simulink model "ejemplo_arduino2"  (R2014b)
settings: Solver=ode3  StartTime=0.0  StopTime=inf  FixedStep=0.001  RelTol=1e-3
libraries: simulink x48, simulink_extras x36, dspswit3 x16, LibrarySimulinkSAS x2, vrlib x2, sldrtlib x1
(part 2 of 2)

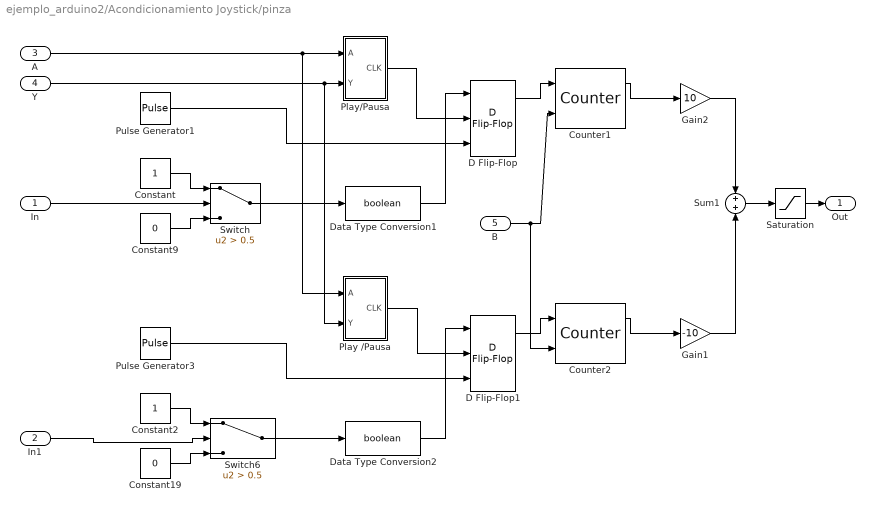
== system ejemplo_arduino2/Acondicionamiento Joystick/pinza ==
  In : Inport
  In1 : Inport  Port=2
  A : Inport  Port=3
  Y : Inport  Port=4
  B : Inport  Port=5
  Constant : Constant
  Constant19 : Constant  Value=0
  Constant2 : Constant
  Constant9 : Constant  Value=0
  Counter1 : dspswit3/Counter  Direction=Up  CountEvent=Rising edge  CounterSize=User defined  MaxCount=255  InitialCount=0  Output=Count and Hit  HitValue=32  ResetInput=on  SamplesPerFrame=1  Ts=1  CntDtype=double  HitDtype=Logical
  Counter2 : dspswit3/Counter  Direction=Up  CountEvent=Rising edge  CounterSize=User defined  MaxCount=255  InitialCount=0  Output=Count and Hit  HitValue=32  ResetInput=on  SamplesPerFrame=1  Ts=1  CntDtype=double  HitDtype=Logical
  D Flip-Flop : simulink_extras/Flip Flops/D Flip-Flop
  D Flip-Flop1 : simulink_extras/Flip Flops/D Flip-Flop
  Data Type Conversion1 : DataTypeConversion  OutDataTypeStr=boolean
  Data Type Conversion2 : DataTypeConversion  OutDataTypeStr=boolean
  Gain1 : Gain  Gain=-10
  Gain2 : Gain  Gain=10
  Play /Pausa : Subsystem
  Play/Pausa : Subsystem
  Pulse Generator1 : DiscretePulseGenerator  PulseType=Time based  Period=0.1  PulseWidth=50
  Pulse Generator3 : DiscretePulseGenerator  PulseType=Time based  Period=0.1  PulseWidth=50
  Saturation : Saturate  UpperLimit=200  LowerLimit=0
  Sum1 : Sum  Inputs=+|+
  Switch : Switch  Criteria=u2 > Threshold  Threshold=0.5  OutDataTypeStr=single  InputSameDT=on
  Switch6 : Switch  Criteria=u2 > Threshold  Threshold=0.5  OutDataTypeStr=single  InputSameDT=on
  Out : Outport
  wires:
  Counter1/1 -> Gain2/1
  Constant/1 -> Switch/1
  Constant9/1 -> Switch/3
  Constant2/1 -> Switch6/1
  Counter2/1 -> Gain1/1
  Gain1/1 -> Sum1/2
  D Flip-Flop1/1 -> Counter2/1
  Switch6/1 -> Data Type Conversion2/1
  Data Type Conversion2/1 -> D Flip-Flop1/1
  Pulse Generator3/1 -> D Flip-Flop1/3
  Constant19/1 -> Switch6/3
  In/1 -> Switch/2
  Saturation/1 -> Out/1
  Pulse Generator1/1 -> D Flip-Flop/3
  Sum1/1 -> Saturation/1
  Gain2/1 -> Sum1/1
  D Flip-Flop/1 -> Counter1/1
  Data Type Conversion1/1 -> D Flip-Flop/1
  Switch/1 -> Data Type Conversion1/1
  In1/1 -> Switch6/2
  Play/Pausa/1(CLK) -> D Flip-Flop/2
  Play /Pausa/1(CLK) -> D Flip-Flop1/2
  A/1 -> Play /Pausa/1(A), Play/Pausa/1(A)
  Y/1 -> Play /Pausa/2(Y), Play/Pausa/2(Y)
  B/1 -> Counter1/2, Counter2/2

== system ejemplo_arduino2/Acondicionamiento Joystick/Horizontal/Play //Pausa ==
  A : Inport
  Y : Inport  Port=2
  Constant1 : Constant  Value=0
  Detect Rise Positive : simulink/Logic and Bit Operations/Detect Rise Positive  vinit=0  InputProcessing=Inherited  OutDataTypeStr=boolean
  Detect Rise Positive1 : simulink/Logic and Bit Operations/Detect Rise Positive  vinit=0  InputProcessing=Inherited  OutDataTypeStr=boolean
  Pulse Generator : DiscretePulseGenerator  PulseType=Time based  Period=0.05  PulseWidth=50
  S-R Flip-Flop : simulink_extras/Flip Flops/S-R Flip-Flop  initial_condition=0
  Switch1 : Switch  Criteria=u2 > Threshold  Threshold=0.5  OutDataTypeStr=single  InputSameDT=on
  CLK : Outport
  wires:
  Pulse Generator/1 -> Switch1/1
  S-R Flip-Flop/1 -> Switch1/2
  Switch1/1 -> CLK/1
  Constant1/1 -> Switch1/3
  Detect Rise Positive1/1 -> S-R Flip-Flop/2
  A/1 -> Detect Rise Positive/1
  Detect Rise Positive/1 -> S-R Flip-Flop/1
  Y/1 -> Detect Rise Positive1/1

== system ejemplo_arduino2/Acondicionamiento Joystick/Horizontal/Play//Pausa ==
  A : Inport
  Y : Inport  Port=2
  Constant1 : Constant  Value=0
  Detect Rise Positive : simulink/Logic and Bit Operations/Detect Rise Positive  vinit=0  InputProcessing=Inherited  OutDataTypeStr=boolean
  Detect Rise Positive1 : simulink/Logic and Bit Operations/Detect Rise Positive  vinit=0  InputProcessing=Inherited  OutDataTypeStr=boolean
  Pulse Generator : DiscretePulseGenerator  PulseType=Time based  Period=0.05  PulseWidth=50
  S-R Flip-Flop : simulink_extras/Flip Flops/S-R Flip-Flop  initial_condition=0
  Switch1 : Switch  Criteria=u2 > Threshold  Threshold=0.5  OutDataTypeStr=single  InputSameDT=on
  CLK : Outport
  wires:
  Pulse Generator/1 -> Switch1/1
  S-R Flip-Flop/1 -> Switch1/2
  Switch1/1 -> CLK/1
  Constant1/1 -> Switch1/3
  Detect Rise Positive1/1 -> S-R Flip-Flop/2
  A/1 -> Detect Rise Positive/1
  Detect Rise Positive/1 -> S-R Flip-Flop/1
  Y/1 -> Detect Rise Positive1/1

== system ejemplo_arduino2/Acondicionamiento Joystick/Vertical/Play //Pausa ==
  A : Inport
  Y : Inport  Port=2
  Constant1 : Constant  Value=0
  Detect Rise Positive : simulink/Logic and Bit Operations/Detect Rise Positive  vinit=0  InputProcessing=Inherited  OutDataTypeStr=boolean
  Detect Rise Positive1 : simulink/Logic and Bit Operations/Detect Rise Positive  vinit=0  InputProcessing=Inherited  OutDataTypeStr=boolean
  Pulse Generator : DiscretePulseGenerator  PulseType=Time based  Period=0.1  PulseWidth=50
  S-R Flip-Flop : simulink_extras/Flip Flops/S-R Flip-Flop  initial_condition=0
  Switch1 : Switch  Criteria=u2 > Threshold  Threshold=0.5  OutDataTypeStr=single  InputSameDT=on
  CLK : Outport
  wires:
  Pulse Generator/1 -> Switch1/1
  S-R Flip-Flop/1 -> Switch1/2
  Switch1/1 -> CLK/1
  Constant1/1 -> Switch1/3
  Detect Rise Positive1/1 -> S-R Flip-Flop/2
  A/1 -> Detect Rise Positive/1
  Detect Rise Positive/1 -> S-R Flip-Flop/1
  Y/1 -> Detect Rise Positive1/1

== system ejemplo_arduino2/Acondicionamiento Joystick/Vertical/Play//Pausa ==
  A : Inport
  Y : Inport  Port=2
  Constant1 : Constant  Value=0
  Detect Rise Positive : simulink/Logic and Bit Operations/Detect Rise Positive  vinit=0  InputProcessing=Inherited  OutDataTypeStr=boolean
  Detect Rise Positive1 : simulink/Logic and Bit Operations/Detect Rise Positive  vinit=0  InputProcessing=Inherited  OutDataTypeStr=boolean
  Pulse Generator : DiscretePulseGenerator  PulseType=Time based  Period=0.1  PulseWidth=50
  S-R Flip-Flop : simulink_extras/Flip Flops/S-R Flip-Flop  initial_condition=0
  Switch1 : Switch  Criteria=u2 > Threshold  Threshold=0.5  OutDataTypeStr=single  InputSameDT=on
  CLK : Outport
  wires:
  Pulse Generator/1 -> Switch1/1
  S-R Flip-Flop/1 -> Switch1/2
  Switch1/1 -> CLK/1
  Constant1/1 -> Switch1/3
  Detect Rise Positive1/1 -> S-R Flip-Flop/2
  A/1 -> Detect Rise Positive/1
  Detect Rise Positive/1 -> S-R Flip-Flop/1
  Y/1 -> Detect Rise Positive1/1

== system ejemplo_arduino2/Acondicionamiento Joystick/mov 1/Play //Pausa ==
  A : Inport
  Y : Inport  Port=2
  Constant1 : Constant  Value=0
  Detect Rise Positive : simulink/Logic and Bit Operations/Detect Rise Positive  vinit=0  InputProcessing=Inherited  OutDataTypeStr=boolean
  Detect Rise Positive1 : simulink/Logic and Bit Operations/Detect Rise Positive  vinit=0  InputProcessing=Inherited  OutDataTypeStr=boolean
  Pulse Generator : DiscretePulseGenerator  PulseType=Time based  Period=0.1  PulseWidth=50
  S-R Flip-Flop : simulink_extras/Flip Flops/S-R Flip-Flop  initial_condition=0
  Switch1 : Switch  Criteria=u2 > Threshold  Threshold=0.5  OutDataTypeStr=single  InputSameDT=on
  CLK : Outport
  wires:
  Pulse Generator/1 -> Switch1/1
  S-R Flip-Flop/1 -> Switch1/2
  Switch1/1 -> CLK/1
  Constant1/1 -> Switch1/3
  Detect Rise Positive1/1 -> S-R Flip-Flop/2
  A/1 -> Detect Rise Positive/1
  Detect Rise Positive/1 -> S-R Flip-Flop/1
  Y/1 -> Detect Rise Positive1/1

== system ejemplo_arduino2/Acondicionamiento Joystick/mov 1/Play//Pausa ==
  A : Inport
  Y : Inport  Port=2
  Constant1 : Constant  Value=0
  Detect Rise Positive : simulink/Logic and Bit Operations/Detect Rise Positive  vinit=0  InputProcessing=Inherited  OutDataTypeStr=boolean
  Detect Rise Positive1 : simulink/Logic and Bit Operations/Detect Rise Positive  vinit=0  InputProcessing=Inherited  OutDataTypeStr=boolean
  Pulse Generator : DiscretePulseGenerator  PulseType=Time based  Period=0.1  PulseWidth=50
  S-R Flip-Flop : simulink_extras/Flip Flops/S-R Flip-Flop  initial_condition=0
  Switch1 : Switch  Criteria=u2 > Threshold  Threshold=0.5  OutDataTypeStr=single  InputSameDT=on
  CLK : Outport
  wires:
  Pulse Generator/1 -> Switch1/1
  S-R Flip-Flop/1 -> Switch1/2
  Switch1/1 -> CLK/1
  Constant1/1 -> Switch1/3
  Detect Rise Positive1/1 -> S-R Flip-Flop/2
  A/1 -> Detect Rise Positive/1
  Detect Rise Positive/1 -> S-R Flip-Flop/1
  Y/1 -> Detect Rise Positive1/1

== system ejemplo_arduino2/Acondicionamiento Joystick/mov 2/Play //Pausa ==
  A : Inport
  Y : Inport  Port=2
  Constant1 : Constant  Value=0
  Detect Rise Positive : simulink/Logic and Bit Operations/Detect Rise Positive  vinit=0  InputProcessing=Inherited  OutDataTypeStr=boolean
  Detect Rise Positive1 : simulink/Logic and Bit Operations/Detect Rise Positive  vinit=0  InputProcessing=Inherited  OutDataTypeStr=boolean
  Pulse Generator : DiscretePulseGenerator  PulseType=Time based  Period=0.1  PulseWidth=50
  S-R Flip-Flop : simulink_extras/Flip Flops/S-R Flip-Flop  initial_condition=0
  Switch1 : Switch  Criteria=u2 > Threshold  Threshold=0.5  OutDataTypeStr=single  InputSameDT=on
  CLK : Outport
  wires:
  Pulse Generator/1 -> Switch1/1
  S-R Flip-Flop/1 -> Switch1/2
  Switch1/1 -> CLK/1
  Constant1/1 -> Switch1/3
  Detect Rise Positive1/1 -> S-R Flip-Flop/2
  A/1 -> Detect Rise Positive/1
  Detect Rise Positive/1 -> S-R Flip-Flop/1
  Y/1 -> Detect Rise Positive1/1

== system ejemplo_arduino2/Acondicionamiento Joystick/mov 2/Play//Pausa ==
  A : Inport
  Y : Inport  Port=2
  Constant1 : Constant  Value=0
  Detect Rise Positive : simulink/Logic and Bit Operations/Detect Rise Positive  vinit=0  InputProcessing=Inherited  OutDataTypeStr=boolean
  Detect Rise Positive1 : simulink/Logic and Bit Operations/Detect Rise Positive  vinit=0  InputProcessing=Inherited  OutDataTypeStr=boolean
  Pulse Generator : DiscretePulseGenerator  PulseType=Time based  Period=0.1  PulseWidth=50
  S-R Flip-Flop : simulink_extras/Flip Flops/S-R Flip-Flop  initial_condition=0
  Switch1 : Switch  Criteria=u2 > Threshold  Threshold=0.5  OutDataTypeStr=single  InputSameDT=on
  CLK : Outport
  wires:
  Pulse Generator/1 -> Switch1/1
  S-R Flip-Flop/1 -> Switch1/2
  Switch1/1 -> CLK/1
  Constant1/1 -> Switch1/3
  Detect Rise Positive1/1 -> S-R Flip-Flop/2
  A/1 -> Detect Rise Positive/1
  Detect Rise Positive/1 -> S-R Flip-Flop/1
  Y/1 -> Detect Rise Positive1/1

== system ejemplo_arduino2/Acondicionamiento Joystick/mov 3/Play //Pausa ==
  A : Inport
  Y : Inport  Port=2
  Constant1 : Constant  Value=0
  Detect Rise Positive : simulink/Logic and Bit Operations/Detect Rise Positive  vinit=0  InputProcessing=Inherited  OutDataTypeStr=boolean
  Detect Rise Positive1 : simulink/Logic and Bit Operations/Detect Rise Positive  vinit=0  InputProcessing=Inherited  OutDataTypeStr=boolean
  Pulse Generator : DiscretePulseGenerator  PulseType=Time based  Period=0.1  PulseWidth=50
  S-R Flip-Flop : simulink_extras/Flip Flops/S-R Flip-Flop  initial_condition=0
  Switch1 : Switch  Criteria=u2 > Threshold  Threshold=0.5  OutDataTypeStr=single  InputSameDT=on
  CLK : Outport
  wires:
  Pulse Generator/1 -> Switch1/1
  S-R Flip-Flop/1 -> Switch1/2
  Switch1/1 -> CLK/1
  Constant1/1 -> Switch1/3
  Detect Rise Positive1/1 -> S-R Flip-Flop/2
  A/1 -> Detect Rise Positive/1
  Detect Rise Positive/1 -> S-R Flip-Flop/1
  Y/1 -> Detect Rise Positive1/1

== system ejemplo_arduino2/Acondicionamiento Joystick/mov 3/Play//Pausa ==
  A : Inport
  Y : Inport  Port=2
  Constant1 : Constant  Value=0
  Detect Rise Positive : simulink/Logic and Bit Operations/Detect Rise Positive  vinit=0  InputProcessing=Inherited  OutDataTypeStr=boolean
  Detect Rise Positive1 : simulink/Logic and Bit Operations/Detect Rise Positive  vinit=0  InputProcessing=Inherited  OutDataTypeStr=boolean
  Pulse Generator : DiscretePulseGenerator  PulseType=Time based  Period=0.1  PulseWidth=50
  S-R Flip-Flop : simulink_extras/Flip Flops/S-R Flip-Flop  initial_condition=0
  Switch1 : Switch  Criteria=u2 > Threshold  Threshold=0.5  OutDataTypeStr=single  InputSameDT=on
  CLK : Outport
  wires:
  Pulse Generator/1 -> Switch1/1
  S-R Flip-Flop/1 -> Switch1/2
  Switch1/1 -> CLK/1
  Constant1/1 -> Switch1/3
  Detect Rise Positive1/1 -> S-R Flip-Flop/2
  A/1 -> Detect Rise Positive/1
  Detect Rise Positive/1 -> S-R Flip-Flop/1
  Y/1 -> Detect Rise Positive1/1

== system ejemplo_arduino2/Acondicionamiento Joystick/mov 4/Play //Pausa ==
  A : Inport
  Y : Inport  Port=2
  Constant1 : Constant  Value=0
  Detect Rise Positive : simulink/Logic and Bit Operations/Detect Rise Positive  vinit=0  InputProcessing=Inherited  OutDataTypeStr=boolean
  Detect Rise Positive1 : simulink/Logic and Bit Operations/Detect Rise Positive  vinit=0  InputProcessing=Inherited  OutDataTypeStr=boolean
  Pulse Generator : DiscretePulseGenerator  PulseType=Time based  Period=0.1  PulseWidth=50
  S-R Flip-Flop : simulink_extras/Flip Flops/S-R Flip-Flop  initial_condition=0
  Switch1 : Switch  Criteria=u2 > Threshold  Threshold=0.5  OutDataTypeStr=single  InputSameDT=on
  CLK : Outport
  wires:
  Pulse Generator/1 -> Switch1/1
  S-R Flip-Flop/1 -> Switch1/2
  Switch1/1 -> CLK/1
  Constant1/1 -> Switch1/3
  Detect Rise Positive1/1 -> S-R Flip-Flop/2
  A/1 -> Detect Rise Positive/1
  Detect Rise Positive/1 -> S-R Flip-Flop/1
  Y/1 -> Detect Rise Positive1/1

== system ejemplo_arduino2/Acondicionamiento Joystick/mov 4/Play//Pausa ==
  A : Inport
  Y : Inport  Port=2
  Constant1 : Constant  Value=0
  Detect Rise Positive : simulink/Logic and Bit Operations/Detect Rise Positive  vinit=0  InputProcessing=Inherited  OutDataTypeStr=boolean
  Detect Rise Positive1 : simulink/Logic and Bit Operations/Detect Rise Positive  vinit=0  InputProcessing=Inherited  OutDataTypeStr=boolean
  Pulse Generator : DiscretePulseGenerator  PulseType=Time based  Period=0.1  PulseWidth=50
  S-R Flip-Flop : simulink_extras/Flip Flops/S-R Flip-Flop  initial_condition=0
  Switch1 : Switch  Criteria=u2 > Threshold  Threshold=0.5  OutDataTypeStr=single  InputSameDT=on
  CLK : Outport
  wires:
  Pulse Generator/1 -> Switch1/1
  S-R Flip-Flop/1 -> Switch1/2
  Switch1/1 -> CLK/1
  Constant1/1 -> Switch1/3
  Detect Rise Positive1/1 -> S-R Flip-Flop/2
  A/1 -> Detect Rise Positive/1
  Detect Rise Positive/1 -> S-R Flip-Flop/1
  Y/1 -> Detect Rise Positive1/1

== system ejemplo_arduino2/Acondicionamiento Joystick/mov 5/Play //Pausa ==
  A : Inport
  Y : Inport  Port=2
  Constant1 : Constant  Value=0
  Detect Rise Positive : simulink/Logic and Bit Operations/Detect Rise Positive  vinit=0  InputProcessing=Inherited  OutDataTypeStr=boolean
  Detect Rise Positive1 : simulink/Logic and Bit Operations/Detect Rise Positive  vinit=0  InputProcessing=Inherited  OutDataTypeStr=boolean
  Pulse Generator : DiscretePulseGenerator  PulseType=Time based  Period=0.1  PulseWidth=50
  S-R Flip-Flop : simulink_extras/Flip Flops/S-R Flip-Flop  initial_condition=0
  Switch1 : Switch  Criteria=u2 > Threshold  Threshold=0.5  OutDataTypeStr=single  InputSameDT=on
  CLK : Outport
  wires:
  Pulse Generator/1 -> Switch1/1
  S-R Flip-Flop/1 -> Switch1/2
  Switch1/1 -> CLK/1
  Constant1/1 -> Switch1/3
  Detect Rise Positive1/1 -> S-R Flip-Flop/2
  A/1 -> Detect Rise Positive/1
  Detect Rise Positive/1 -> S-R Flip-Flop/1
  Y/1 -> Detect Rise Positive1/1

== system ejemplo_arduino2/Acondicionamiento Joystick/mov 5/Play//Pausa ==
  A : Inport
  Y : Inport  Port=2
  Constant1 : Constant  Value=0
  Detect Rise Positive : simulink/Logic and Bit Operations/Detect Rise Positive  vinit=0  InputProcessing=Inherited  OutDataTypeStr=boolean
  Detect Rise Positive1 : simulink/Logic and Bit Operations/Detect Rise Positive  vinit=0  InputProcessing=Inherited  OutDataTypeStr=boolean
  Pulse Generator : DiscretePulseGenerator  PulseType=Time based  Period=0.1  PulseWidth=50
  S-R Flip-Flop : simulink_extras/Flip Flops/S-R Flip-Flop  initial_condition=0
  Switch1 : Switch  Criteria=u2 > Threshold  Threshold=0.5  OutDataTypeStr=single  InputSameDT=on
  CLK : Outport
  wires:
  Pulse Generator/1 -> Switch1/1
  S-R Flip-Flop/1 -> Switch1/2
  Switch1/1 -> CLK/1
  Constant1/1 -> Switch1/3
  Detect Rise Positive1/1 -> S-R Flip-Flop/2
  A/1 -> Detect Rise Positive/1
  Detect Rise Positive/1 -> S-R Flip-Flop/1
  Y/1 -> Detect Rise Positive1/1

== system ejemplo_arduino2/Acondicionamiento Joystick/pinza/Play //Pausa ==
  A : Inport
  Y : Inport  Port=2
  Constant1 : Constant  Value=0
  Detect Rise Positive : simulink/Logic and Bit Operations/Detect Rise Positive  vinit=0  InputProcessing=Inherited  OutDataTypeStr=boolean
  Detect Rise Positive1 : simulink/Logic and Bit Operations/Detect Rise Positive  vinit=0  InputProcessing=Inherited  OutDataTypeStr=boolean
  Pulse Generator : DiscretePulseGenerator  PulseType=Time based  Period=0.1  PulseWidth=50
  S-R Flip-Flop : simulink_extras/Flip Flops/S-R Flip-Flop  initial_condition=0
  Switch1 : Switch  Criteria=u2 > Threshold  Threshold=0.5  OutDataTypeStr=single  InputSameDT=on
  CLK : Outport
  wires:
  Pulse Generator/1 -> Switch1/1
  S-R Flip-Flop/1 -> Switch1/2
  Switch1/1 -> CLK/1
  Constant1/1 -> Switch1/3
  Detect Rise Positive1/1 -> S-R Flip-Flop/2
  A/1 -> Detect Rise Positive/1
  Detect Rise Positive/1 -> S-R Flip-Flop/1
  Y/1 -> Detect Rise Positive1/1

== system ejemplo_arduino2/Acondicionamiento Joystick/pinza/Play//Pausa ==
  A : Inport
  Y : Inport  Port=2
  Constant1 : Constant  Value=0
  Detect Rise Positive : simulink/Logic and Bit Operations/Detect Rise Positive  vinit=0  InputProcessing=Inherited  OutDataTypeStr=boolean
  Detect Rise Positive1 : simulink/Logic and Bit Operations/Detect Rise Positive  vinit=0  InputProcessing=Inherited  OutDataTypeStr=boolean
  Pulse Generator : DiscretePulseGenerator  PulseType=Time based  Period=0.1  PulseWidth=50
  S-R Flip-Flop : simulink_extras/Flip Flops/S-R Flip-Flop  initial_condition=0
  Switch1 : Switch  Criteria=u2 > Threshold  Threshold=0.5  OutDataTypeStr=single  InputSameDT=on
  CLK : Outport
  wires:
  Pulse Generator/1 -> Switch1/1
  S-R Flip-Flop/1 -> Switch1/2
  Switch1/1 -> CLK/1
  Constant1/1 -> Switch1/3
  Detect Rise Positive1/1 -> S-R Flip-Flop/2
  A/1 -> Detect Rise Positive/1
  Detect Rise Positive/1 -> S-R Flip-Flop/1
  Y/1 -> Detect Rise Positive1/1
